simulink model "Model_V5"  (R2024b)
settings: Solver=VariableStepAuto  StartTime=0.0  StopTime=3600*12  RelTol=1e-3
undefined symbols (not defined in the file): PropsSI
libraries: fl_lib x569, SimscapeFluids_lib x61, nesl_utility x27
(part 6 of 7)

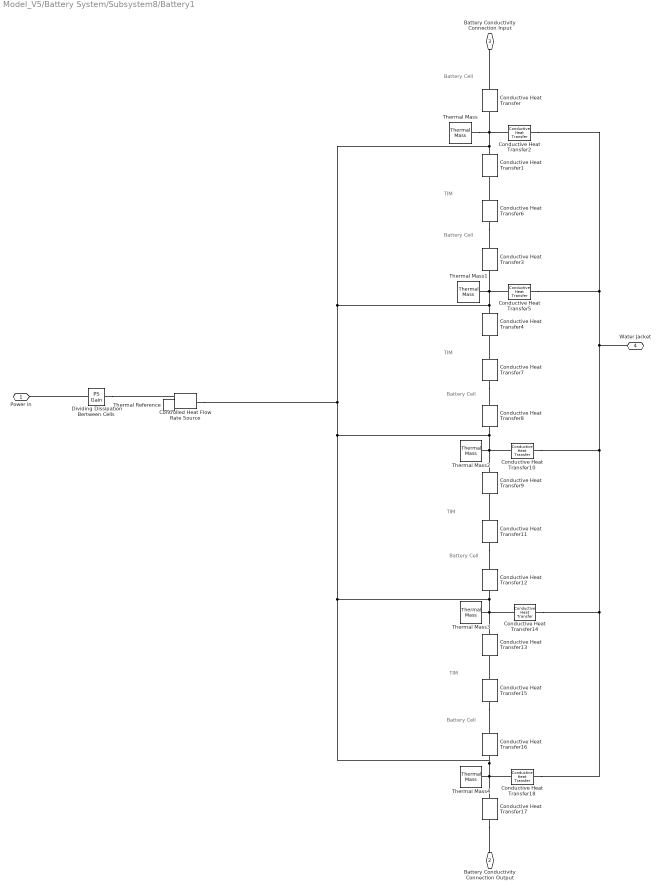
== system Model_V5/Battery System/Subsystem8/Battery1 ==
  note: TIM
  note: Battery Cell
  note: TIM
  note: Battery Cell
  note: TIM
  note: Battery Cell
  note: TIM
  note: Battery Cell
  note: Battery Cell
  Conductive Heat Transfer{,1,3..4,8..9,12..13,16..17} (10 alike) : fl_lib/Thermal/Thermal Elements/Conductive Heat Transfer  thermal_type=foundation.enum.ConstantVariableTabulated.Constant  wall_geometry=foundation.enum.ConductionWallGeometry.Planar  area=301.5*99.7 mm^2  thickness=11.6/2 mm  d_in=0.05 m  d_out=0.1 m  L=1 m  th_cond_min=10 W/(K*m)  th_cond=19 W/(K*m)  th_cond_TLU=[413, 401, 392, 383, 371, 357, 342] W/(K*m)  temp_TLU=[200, 273, 400, 600, 800, 1000, 1200] K  T_specify=off  T_priority=None  T=0 K  T_nominal_specify=off  T_nominal_value=1  T_nominal_unit=K  Q_specify=off  Q_priority=None  Q=0 W  Q_nominal_specify=off  Q_nominal_value=1  Q_nominal_unit=W
  Conductive Heat Transfer{2,5,10,14,18} (5 alike) : fl_lib/Thermal/Thermal Elements/Conductive Heat Transfer  thermal_type=foundation.enum.ConstantVariableTabulated.Constant  wall_geometry=foundation.enum.ConductionWallGeometry.Planar  area=(2*(301.1*11.6)) + (2*(99.9*11.7)) mm^2  thickness=0.003 in  d_in=0.05 m  d_out=0.1 m  L=1 m  th_cond_min=10 W/(K*m)  th_cond=1.38 W/(K*m)  th_cond_TLU=[413, 401, 392, 383, 371, 357, 342] W/(K*m)  temp_TLU=[200, 273, 400, 600, 800, 1000, 1200] K  T_specify=off  T_priority=None  T=0 K  T_nominal_specify=off  T_nominal_value=1  T_nominal_unit=K  Q_specify=off  Q_priority=None  Q=0 W  Q_nominal_specify=off  Q_nominal_value=1  Q_nominal_unit=W
  Conductive Heat Transfer{6..7,11,15} (4 alike) : fl_lib/Thermal/Thermal Elements/Conductive Heat Transfer  thermal_type=foundation.enum.ConstantVariableTabulated.Constant  wall_geometry=foundation.enum.ConductionWallGeometry.Planar  area=301.5*99.7 mm^2  thickness=0.003 in  d_in=0.05 m  d_out=0.1 m  L=1 m  th_cond_min=10 W/(K*m)  th_cond=8.89 W/(K*m)  th_cond_TLU=[413, 401, 392, 383, 371, 357, 342] W/(K*m)  temp_TLU=[200, 273, 400, 600, 800, 1000, 1200] K  T_specify=off  T_priority=None  T=0 K  T_nominal_specify=off  T_nominal_value=1  T_nominal_unit=K  Q_specify=off  Q_priority=None  Q=0 W  Q_nominal_specify=off  Q_nominal_value=1  Q_nominal_unit=W
  Controlled Heat Flow Rate Source : fl_lib/Thermal/Thermal Sources/Controlled Heat Flow Rate Source
  Dividing Dissipation Bertween Cells : fl_lib/Physical Signals/Functions/PS Gain  gain=1/5
  Thermal Mass{,1..4} (5 alike) : fl_lib/Thermal/Thermal Elements/Thermal Mass  mass_type=foundation.enum.constant_variable.constant  mass=740 g  sp_heat=1040 J/(K*kg)  mass_min=1e-6 kg  num_ports=foundation.enum.numPorts2.one  m_specify=off  m_priority=High  m=1 kg  m_nominal_specify=off  m_nominal_value=1  m_nominal_unit=kg  T_specify=on  T_priority=Low  T=292 K  T_nominal_specify=off  T_nominal_value=1  T_nominal_unit=K  Q_specify=off  Q_priority=None  Q=0 W  Q_nominal_specify=off  Q_nominal_value=1  Q_nominal_unit=W
  Thermal Reference : fl_lib/Thermal/Thermal Elements/Thermal Reference
  Power in : PMIOPort  Side=Left
  Battery Conductivity Connection Output : PMIOPort  Port=2  Side=Left
  Battery Conductivity Connection Input : PMIOPort  Port=3  Side=Right
  Water Jacket : PMIOPort  Port=4  Side=Right
  connections:
  Conductive Heat Transfer7/RConn1 -- Conductive Heat Transfer8/LConn1
  Conductive Heat Transfer17/RConn1 -- Battery Conductivity Connection Output/RConn1
  Conductive Heat Transfer6/RConn1 -- Conductive Heat Transfer3/LConn1
  Conductive Heat Transfer18/RConn1 -- Conductive Heat Transfer14/RConn1 -- Conductive Heat Transfer10/RConn1 -- Conductive Heat Transfer2/RConn1 -- Conductive Heat Transfer5/RConn1 -- Water Jacket/RConn1
  Conductive Heat Transfer8/RConn1 -- Conductive Heat Transfer10/LConn1 -- Thermal Mass2/LConn1 -- Conductive Heat Transfer9/LConn1 -- Conductive Heat Transfer12/RConn1 -- Thermal Mass3/LConn1 -- Conductive Heat Transfer14/LConn1 -- Conductive Heat Transfer13/LConn1 -- Conductive Heat Transfer18/LConn1 -- Thermal Mass4/LConn1 -- Conductive Heat Transfer17/LConn1 -- Conductive Heat Transfer16/RConn1 -- Conductive Heat Transfer2/LConn1 -- Thermal Mass/LConn1 -- Conductive Heat Transfer/RConn1 -- Conductive Heat Transfer1/LConn1 -- Conductive Heat Transfer5/LConn1 -- Thermal Mass1/LConn1 -- Conductive Heat Transfer3/RConn1 -- Conductive Heat Transfer4/LConn1 -- Controlled Heat Flow Rate Source/LConn1
  Conductive Heat Transfer15/LConn1 -- Conductive Heat Transfer13/RConn1
  Conductive Heat Transfer11/LConn1 -- Conductive Heat Transfer9/RConn1
  Conductive Heat Transfer7/LConn1 -- Conductive Heat Transfer4/RConn1
  Conductive Heat Transfer11/RConn1 -- Conductive Heat Transfer12/LConn1
  Conductive Heat Transfer6/LConn1 -- Conductive Heat Transfer1/RConn1
  Conductive Heat Transfer15/RConn1 -- Conductive Heat Transfer16/LConn1
  Conductive Heat Transfer/LConn1 -- Battery Conductivity Connection Input/RConn1
  Thermal Reference/LConn1 -- Controlled Heat Flow Rate Source/RConn2
  Dividing Dissipation Bertween Cells/LConn1 -- Power in/RConn1
  Dividing Dissipation Bertween Cells/RConn1 -- Controlled Heat Flow Rate Source/RConn1

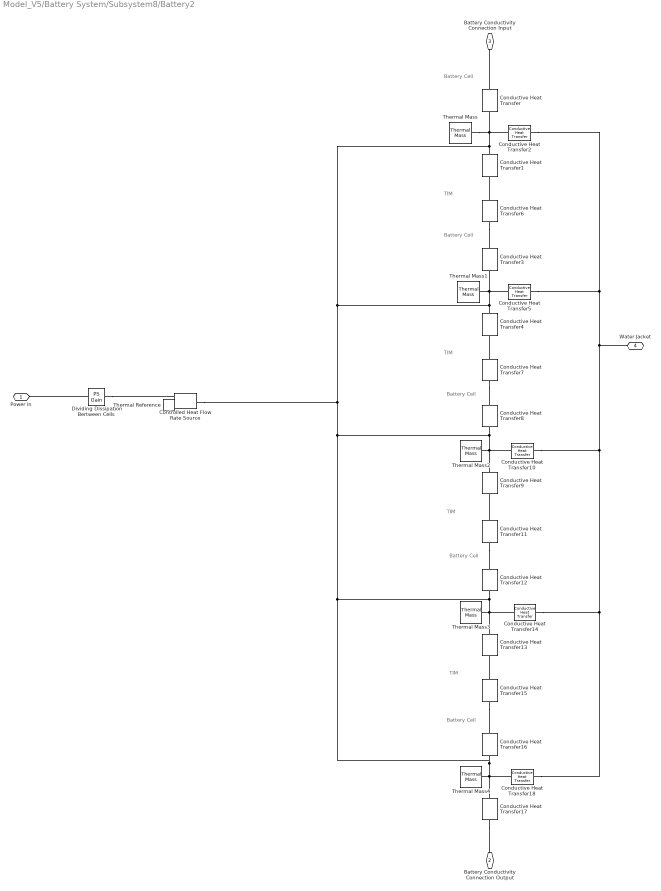
== system Model_V5/Battery System/Subsystem8/Battery2 ==
  note: TIM
  note: Battery Cell
  note: TIM
  note: Battery Cell
  note: TIM
  note: Battery Cell
  note: TIM
  note: Battery Cell
  note: Battery Cell
  Conductive Heat Transfer{,1,3..4,8..9,12..13,16..17} (10 alike) : fl_lib/Thermal/Thermal Elements/Conductive Heat Transfer  thermal_type=foundation.enum.ConstantVariableTabulated.Constant  wall_geometry=foundation.enum.ConductionWallGeometry.Planar  area=301.5*99.7 mm^2  thickness=11.6/2 mm  d_in=0.05 m  d_out=0.1 m  L=1 m  th_cond_min=10 W/(K*m)  th_cond=19 W/(K*m)  th_cond_TLU=[413, 401, 392, 383, 371, 357, 342] W/(K*m)  temp_TLU=[200, 273, 400, 600, 800, 1000, 1200] K  T_specify=off  T_priority=None  T=0 K  T_nominal_specify=off  T_nominal_value=1  T_nominal_unit=K  Q_specify=off  Q_priority=None  Q=0 W  Q_nominal_specify=off  Q_nominal_value=1  Q_nominal_unit=W
  Conductive Heat Transfer{2,5,10,14,18} (5 alike) : fl_lib/Thermal/Thermal Elements/Conductive Heat Transfer  thermal_type=foundation.enum.ConstantVariableTabulated.Constant  wall_geometry=foundation.enum.ConductionWallGeometry.Planar  area=(2*(301.1*11.6)) + (2*(99.9*11.7)) mm^2  thickness=0.003 in  d_in=0.05 m  d_out=0.1 m  L=1 m  th_cond_min=10 W/(K*m)  th_cond=1.38 W/(K*m)  th_cond_TLU=[413, 401, 392, 383, 371, 357, 342] W/(K*m)  temp_TLU=[200, 273, 400, 600, 800, 1000, 1200] K  T_specify=off  T_priority=None  T=0 K  T_nominal_specify=off  T_nominal_value=1  T_nominal_unit=K  Q_specify=off  Q_priority=None  Q=0 W  Q_nominal_specify=off  Q_nominal_value=1  Q_nominal_unit=W
  Conductive Heat Transfer{6..7,11,15} (4 alike) : fl_lib/Thermal/Thermal Elements/Conductive Heat Transfer  thermal_type=foundation.enum.ConstantVariableTabulated.Constant  wall_geometry=foundation.enum.ConductionWallGeometry.Planar  area=301.5*99.7 mm^2  thickness=0.003 in  d_in=0.05 m  d_out=0.1 m  L=1 m  th_cond_min=10 W/(K*m)  th_cond=8.89 W/(K*m)  th_cond_TLU=[413, 401, 392, 383, 371, 357, 342] W/(K*m)  temp_TLU=[200, 273, 400, 600, 800, 1000, 1200] K  T_specify=off  T_priority=None  T=0 K  T_nominal_specify=off  T_nominal_value=1  T_nominal_unit=K  Q_specify=off  Q_priority=None  Q=0 W  Q_nominal_specify=off  Q_nominal_value=1  Q_nominal_unit=W
  Controlled Heat Flow Rate Source : fl_lib/Thermal/Thermal Sources/Controlled Heat Flow Rate Source
  Dividing Dissipation Bertween Cells : fl_lib/Physical Signals/Functions/PS Gain  gain=1/5
  Thermal Mass{,1..4} (5 alike) : fl_lib/Thermal/Thermal Elements/Thermal Mass  mass_type=foundation.enum.constant_variable.constant  mass=740 g  sp_heat=1040 J/(K*kg)  mass_min=1e-6 kg  num_ports=foundation.enum.numPorts2.one  m_specify=off  m_priority=High  m=1 kg  m_nominal_specify=off  m_nominal_value=1  m_nominal_unit=kg  T_specify=on  T_priority=Low  T=292 K  T_nominal_specify=off  T_nominal_value=1  T_nominal_unit=K  Q_specify=off  Q_priority=None  Q=0 W  Q_nominal_specify=off  Q_nominal_value=1  Q_nominal_unit=W
  Thermal Reference : fl_lib/Thermal/Thermal Elements/Thermal Reference
  Power in : PMIOPort  Side=Left
  Battery Conductivity Connection Output : PMIOPort  Port=2  Side=Left
  Battery Conductivity Connection Input : PMIOPort  Port=3  Side=Right
  Water Jacket : PMIOPort  Port=4  Side=Right
  connections:
  Conductive Heat Transfer7/RConn1 -- Conductive Heat Transfer8/LConn1
  Conductive Heat Transfer17/RConn1 -- Battery Conductivity Connection Output/RConn1
  Conductive Heat Transfer6/RConn1 -- Conductive Heat Transfer3/LConn1
  Conductive Heat Transfer18/RConn1 -- Conductive Heat Transfer14/RConn1 -- Conductive Heat Transfer10/RConn1 -- Conductive Heat Transfer2/RConn1 -- Conductive Heat Transfer5/RConn1 -- Water Jacket/RConn1
  Conductive Heat Transfer8/RConn1 -- Conductive Heat Transfer10/LConn1 -- Thermal Mass2/LConn1 -- Conductive Heat Transfer9/LConn1 -- Conductive Heat Transfer12/RConn1 -- Thermal Mass3/LConn1 -- Conductive Heat Transfer14/LConn1 -- Conductive Heat Transfer13/LConn1 -- Conductive Heat Transfer18/LConn1 -- Thermal Mass4/LConn1 -- Conductive Heat Transfer17/LConn1 -- Conductive Heat Transfer16/RConn1 -- Conductive Heat Transfer2/LConn1 -- Thermal Mass/LConn1 -- Conductive Heat Transfer/RConn1 -- Conductive Heat Transfer1/LConn1 -- Conductive Heat Transfer5/LConn1 -- Thermal Mass1/LConn1 -- Conductive Heat Transfer3/RConn1 -- Conductive Heat Transfer4/LConn1 -- Controlled Heat Flow Rate Source/LConn1
  Conductive Heat Transfer15/LConn1 -- Conductive Heat Transfer13/RConn1
  Conductive Heat Transfer11/LConn1 -- Conductive Heat Transfer9/RConn1
  Conductive Heat Transfer7/LConn1 -- Conductive Heat Transfer4/RConn1
  Conductive Heat Transfer11/RConn1 -- Conductive Heat Transfer12/LConn1
  Conductive Heat Transfer6/LConn1 -- Conductive Heat Transfer1/RConn1
  Conductive Heat Transfer15/RConn1 -- Conductive Heat Transfer16/LConn1
  Conductive Heat Transfer/LConn1 -- Battery Conductivity Connection Input/RConn1
  Thermal Reference/LConn1 -- Controlled Heat Flow Rate Source/RConn2
  Dividing Dissipation Bertween Cells/LConn1 -- Power in/RConn1
  Dividing Dissipation Bertween Cells/RConn1 -- Controlled Heat Flow Rate Source/RConn1

== system Model_V5/Battery System/Subsystem8/Battery3 ==
  note: TIM
  note: Battery Cell
  note: TIM
  note: Battery Cell
  note: TIM
  note: Battery Cell
  note: TIM
  note: Battery Cell
  note: Battery Cell
  Conductive Heat Transfer{,1,3..4,8..9,12..13,16} (9 alike) : fl_lib/Thermal/Thermal Elements/Conductive Heat Transfer  thermal_type=foundation.enum.ConstantVariableTabulated.Constant  wall_geometry=foundation.enum.ConductionWallGeometry.Planar  area=301.5*99.7 mm^2  thickness=11.6/2 mm  d_in=0.05 m  d_out=0.1 m  L=1 m  th_cond_min=10 W/(K*m)  th_cond=19 W/(K*m)  th_cond_TLU=[413, 401, 392, 383, 371, 357, 342] W/(K*m)  temp_TLU=[200, 273, 400, 600, 800, 1000, 1200] K  T_specify=off  T_priority=None  T=0 K  T_nominal_specify=off  T_nominal_value=1  T_nominal_unit=K  Q_specify=off  Q_priority=None  Q=0 W  Q_nominal_specify=off  Q_nominal_value=1  Q_nominal_unit=W
  Conductive Heat Transfer{2,5,10,14,18} (5 alike) : fl_lib/Thermal/Thermal Elements/Conductive Heat Transfer  thermal_type=foundation.enum.ConstantVariableTabulated.Constant  wall_geometry=foundation.enum.ConductionWallGeometry.Planar  area=(2*(301.1*11.6)) + (2*(99.9*11.7)) mm^2  thickness=0.003 in  d_in=0.05 m  d_out=0.1 m  L=1 m  th_cond_min=10 W/(K*m)  th_cond=1.38 W/(K*m)  th_cond_TLU=[413, 401, 392, 383, 371, 357, 342] W/(K*m)  temp_TLU=[200, 273, 400, 600, 800, 1000, 1200] K  T_specify=off  T_priority=None  T=0 K  T_nominal_specify=off  T_nominal_value=1  T_nominal_unit=K  Q_specify=off  Q_priority=None  Q=0 W  Q_nominal_specify=off  Q_nominal_value=1  Q_nominal_unit=W
  Conductive Heat Transfer{6..7,11,15} (4 alike) : fl_lib/Thermal/Thermal Elements/Conductive Heat Transfer  thermal_type=foundation.enum.ConstantVariableTabulated.Constant  wall_geometry=foundation.enum.ConductionWallGeometry.Planar  area=301.5*99.7 mm^2  thickness=0.003 in  d_in=0.05 m  d_out=0.1 m  L=1 m  th_cond_min=10 W/(K*m)  th_cond=8.89 W/(K*m)  th_cond_TLU=[413, 401, 392, 383, 371, 357, 342] W/(K*m)  temp_TLU=[200, 273, 400, 600, 800, 1000, 1200] K  T_specify=off  T_priority=None  T=0 K  T_nominal_specify=off  T_nominal_value=1  T_nominal_unit=K  Q_specify=off  Q_priority=None  Q=0 W  Q_nominal_specify=off  Q_nominal_value=1  Q_nominal_unit=W
  Controlled Heat Flow Rate Source : fl_lib/Thermal/Thermal Sources/Controlled Heat Flow Rate Source
  Dividing Dissipation Bertween Cells : fl_lib/Physical Signals/Functions/PS Gain  gain=1/5
  Thermal Mass{,1..4} (5 alike) : fl_lib/Thermal/Thermal Elements/Thermal Mass  mass_type=foundation.enum.constant_variable.constant  mass=740 g  sp_heat=1040 J/(K*kg)  mass_min=1e-6 kg  num_ports=foundation.enum.numPorts2.one  m_specify=off  m_priority=High  m=1 kg  m_nominal_specify=off  m_nominal_value=1  m_nominal_unit=kg  T_specify=on  T_priority=Low  T=292 K  T_nominal_specify=off  T_nominal_value=1  T_nominal_unit=K  Q_specify=off  Q_priority=None  Q=0 W  Q_nominal_specify=off  Q_nominal_value=1  Q_nominal_unit=W
  Thermal Reference : fl_lib/Thermal/Thermal Elements/Thermal Reference
  Power in : PMIOPort  Side=Left
  Battery Conductivity Connection Input : PMIOPort  Port=2  Side=Right
  Water Jacket : PMIOPort  Port=3  Side=Right
  connections:
  Conductive Heat Transfer7/RConn1 -- Conductive Heat Transfer8/LConn1
  Conductive Heat Transfer6/RConn1 -- Conductive Heat Transfer3/LConn1
  Conductive Heat Transfer18/RConn1 -- Conductive Heat Transfer14/RConn1 -- Conductive Heat Transfer10/RConn1 -- Conductive Heat Transfer2/RConn1 -- Conductive Heat Transfer5/RConn1 -- Water Jacket/RConn1
  Conductive Heat Transfer8/RConn1 -- Conductive Heat Transfer10/LConn1 -- Thermal Mass2/LConn1 -- Conductive Heat Transfer9/LConn1 -- Conductive Heat Transfer12/RConn1 -- Thermal Mass3/LConn1 -- Conductive Heat Transfer14/LConn1 -- Conductive Heat Transfer13/LConn1 -- Conductive Heat Transfer18/LConn1 -- Thermal Mass4/LConn1 -- Conductive Heat Transfer16/RConn1 -- Conductive Heat Transfer2/LConn1 -- Thermal Mass/LConn1 -- Conductive Heat Transfer/RConn1 -- Conductive Heat Transfer1/LConn1 -- Conductive Heat Transfer5/LConn1 -- Thermal Mass1/LConn1 -- Conductive Heat Transfer3/RConn1 -- Conductive Heat Transfer4/LConn1 -- Controlled Heat Flow Rate Source/LConn1
  Conductive Heat Transfer15/LConn1 -- Conductive Heat Transfer13/RConn1
  Conductive Heat Transfer11/LConn1 -- Conductive Heat Transfer9/RConn1
  Conductive Heat Transfer7/LConn1 -- Conductive Heat Transfer4/RConn1
  Conductive Heat Transfer11/RConn1 -- Conductive Heat Transfer12/LConn1
  Conductive Heat Transfer6/LConn1 -- Conductive Heat Transfer1/RConn1
  Conductive Heat Transfer15/RConn1 -- Conductive Heat Transfer16/LConn1
  Conductive Heat Transfer/LConn1 -- Battery Conductivity Connection Input/RConn1
  Thermal Reference/LConn1 -- Controlled Heat Flow Rate Source/RConn2
  Dividing Dissipation Bertween Cells/LConn1 -- Power in/RConn1
  Dividing Dissipation Bertween Cells/RConn1 -- Controlled Heat Flow Rate Source/RConn1

== system Model_V5/Battery System/Subsystem8/Battery4 ==
  note: TIM
  note: Battery Cell
  note: TIM
  note: Battery Cell
  note: TIM
  note: Battery Cell
  note: TIM
  note: Battery Cell
  note: Battery Cell
  Conductive Heat Transfer{1,3..4,8..9,12..13,16..17} (9 alike) : fl_lib/Thermal/Thermal Elements/Conductive Heat Transfer  thermal_type=foundation.enum.ConstantVariableTabulated.Constant  wall_geometry=foundation.enum.ConductionWallGeometry.Planar  area=301.5*99.7 mm^2  thickness=11.6/2 mm  d_in=0.05 m  d_out=0.1 m  L=1 m  th_cond_min=10 W/(K*m)  th_cond=19 W/(K*m)  th_cond_TLU=[413, 401, 392, 383, 371, 357, 342] W/(K*m)  temp_TLU=[200, 273, 400, 600, 800, 1000, 1200] K  T_specify=off  T_priority=None  T=0 K  T_nominal_specify=off  T_nominal_value=1  T_nominal_unit=K  Q_specify=off  Q_priority=None  Q=0 W  Q_nominal_specify=off  Q_nominal_value=1  Q_nominal_unit=W
  Conductive Heat Transfer{2,5,10,14,18} (5 alike) : fl_lib/Thermal/Thermal Elements/Conductive Heat Transfer  thermal_type=foundation.enum.ConstantVariableTabulated.Constant  wall_geometry=foundation.enum.ConductionWallGeometry.Planar  area=(2*(301.1*11.6)) + (2*(99.9*11.7)) mm^2  thickness=0.003 in  d_in=0.05 m  d_out=0.1 m  L=1 m  th_cond_min=10 W/(K*m)  th_cond=1.38 W/(K*m)  th_cond_TLU=[413, 401, 392, 383, 371, 357, 342] W/(K*m)  temp_TLU=[200, 273, 400, 600, 800, 1000, 1200] K  T_specify=off  T_priority=None  T=0 K  T_nominal_specify=off  T_nominal_value=1  T_nominal_unit=K  Q_specify=off  Q_priority=None  Q=0 W  Q_nominal_specify=off  Q_nominal_value=1  Q_nominal_unit=W
  Conductive Heat Transfer{6..7,11,15} (4 alike) : fl_lib/Thermal/Thermal Elements/Conductive Heat Transfer  thermal_type=foundation.enum.ConstantVariableTabulated.Constant  wall_geometry=foundation.enum.ConductionWallGeometry.Planar  area=301.5*99.7 mm^2  thickness=0.003 in  d_in=0.05 m  d_out=0.1 m  L=1 m  th_cond_min=10 W/(K*m)  th_cond=8.89 W/(K*m)  th_cond_TLU=[413, 401, 392, 383, 371, 357, 342] W/(K*m)  temp_TLU=[200, 273, 400, 600, 800, 1000, 1200] K  T_specify=off  T_priority=None  T=0 K  T_nominal_specify=off  T_nominal_value=1  T_nominal_unit=K  Q_specify=off  Q_priority=None  Q=0 W  Q_nominal_specify=off  Q_nominal_value=1  Q_nominal_unit=W
  Controlled Heat Flow Rate Source : fl_lib/Thermal/Thermal Sources/Controlled Heat Flow Rate Source
  Dividing Dissipation Bertween Cells : fl_lib/Physical Signals/Functions/PS Gain  gain=1/5
  Thermal Mass{,1..4} (5 alike) : fl_lib/Thermal/Thermal Elements/Thermal Mass  mass_type=foundation.enum.constant_variable.constant  mass=740 g  sp_heat=1040 J/(K*kg)  mass_min=1e-6 kg  num_ports=foundation.enum.numPorts2.one  m_specify=off  m_priority=High  m=1 kg  m_nominal_specify=off  m_nominal_value=1  m_nominal_unit=kg  T_specify=on  T_priority=Low  T=292 K  T_nominal_specify=off  T_nominal_value=1  T_nominal_unit=K  Q_specify=off  Q_priority=None  Q=0 W  Q_nominal_specify=off  Q_nominal_value=1  Q_nominal_unit=W
  Thermal Reference : fl_lib/Thermal/Thermal Elements/Thermal Reference
  Power in : PMIOPort  Side=Left
  Water Jacket : PMIOPort  Port=2  Side=Right
  Battery Conductivity Connection Output : PMIOPort  Port=3  Side=Right
  connections:
  Conductive Heat Transfer7/RConn1 -- Conductive Heat Transfer8/LConn1
  Conductive Heat Transfer17/RConn1 -- Battery Conductivity Connection Output/RConn1
  Conductive Heat Transfer6/RConn1 -- Conductive Heat Transfer3/LConn1
  Conductive Heat Transfer18/RConn1 -- Conductive Heat Transfer14/RConn1 -- Conductive Heat Transfer10/RConn1 -- Conductive Heat Transfer2/RConn1 -- Conductive Heat Transfer5/RConn1 -- Water Jacket/RConn1
  Conductive Heat Transfer8/RConn1 -- Conductive Heat Transfer10/LConn1 -- Thermal Mass2/LConn1 -- Conductive Heat Transfer9/LConn1 -- Conductive Heat Transfer12/RConn1 -- Thermal Mass3/LConn1 -- Conductive Heat Transfer14/LConn1 -- Conductive Heat Transfer13/LConn1 -- Conductive Heat Transfer18/LConn1 -- Thermal Mass4/LConn1 -- Conductive Heat Transfer17/LConn1 -- Conductive Heat Transfer16/RConn1 -- Conductive Heat Transfer2/LConn1 -- Thermal Mass/LConn1 -- Conductive Heat Transfer1/LConn1 -- Conductive Heat Transfer5/LConn1 -- Thermal Mass1/LConn1 -- Conductive Heat Transfer3/RConn1 -- Conductive Heat Transfer4/LConn1 -- Controlled Heat Flow Rate Source/LConn1
  Conductive Heat Transfer15/LConn1 -- Conductive Heat Transfer13/RConn1
  Conductive Heat Transfer11/LConn1 -- Conductive Heat Transfer9/RConn1
  Conductive Heat Transfer7/LConn1 -- Conductive Heat Transfer4/RConn1
  Conductive Heat Transfer11/RConn1 -- Conductive Heat Transfer12/LConn1
  Conductive Heat Transfer6/LConn1 -- Conductive Heat Transfer1/RConn1
  Conductive Heat Transfer15/RConn1 -- Conductive Heat Transfer16/LConn1
  Thermal Reference/LConn1 -- Controlled Heat Flow Rate Source/RConn2
  Dividing Dissipation Bertween Cells/LConn1 -- Power in/RConn1
  Dividing Dissipation Bertween Cells/RConn1 -- Controlled Heat Flow Rate Source/RConn1

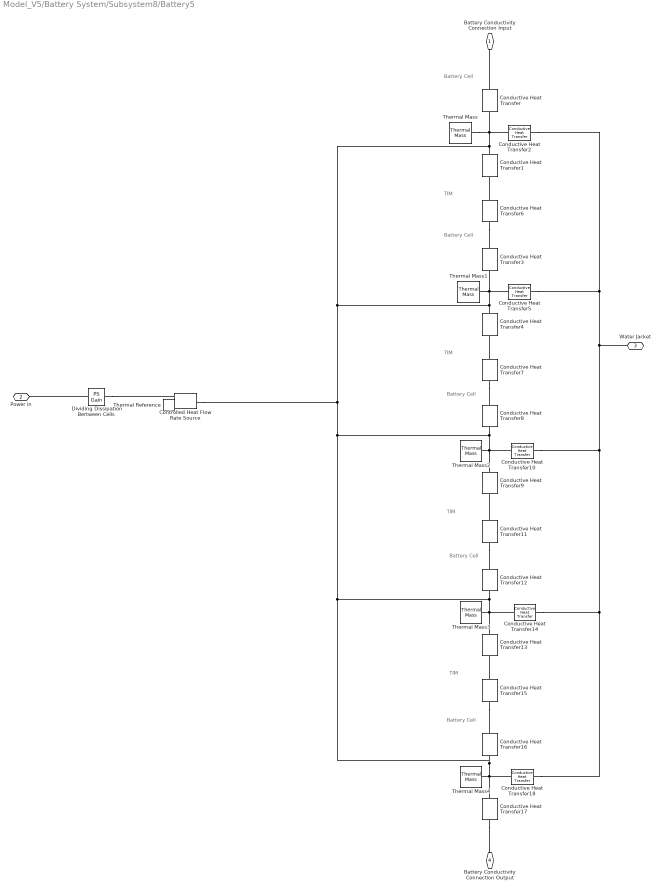
== system Model_V5/Battery System/Subsystem8/Battery5 ==
  note: TIM
  note: Battery Cell
  note: TIM
  note: Battery Cell
  note: TIM
  note: Battery Cell
  note: TIM
  note: Battery Cell
  note: Battery Cell
  Conductive Heat Transfer{,1,3..4,8..9,12..13,16..17} (10 alike) : fl_lib/Thermal/Thermal Elements/Conductive Heat Transfer  thermal_type=foundation.enum.ConstantVariableTabulated.Constant  wall_geometry=foundation.enum.ConductionWallGeometry.Planar  area=301.5*99.7 mm^2  thickness=11.6/2 mm  d_in=0.05 m  d_out=0.1 m  L=1 m  th_cond_min=10 W/(K*m)  th_cond=19 W/(K*m)  th_cond_TLU=[413, 401, 392, 383, 371, 357, 342] W/(K*m)  temp_TLU=[200, 273, 400, 600, 800, 1000, 1200] K  T_specify=off  T_priority=None  T=0 K  T_nominal_specify=off  T_nominal_value=1  T_nominal_unit=K  Q_specify=off  Q_priority=None  Q=0 W  Q_nominal_specify=off  Q_nominal_value=1  Q_nominal_unit=W
  Conductive Heat Transfer{2,5,10,14,18} (5 alike) : fl_lib/Thermal/Thermal Elements/Conductive Heat Transfer  thermal_type=foundation.enum.ConstantVariableTabulated.Constant  wall_geometry=foundation.enum.ConductionWallGeometry.Planar  area=(2*(301.1*11.6)) + (2*(99.9*11.7)) mm^2  thickness=0.003 in  d_in=0.05 m  d_out=0.1 m  L=1 m  th_cond_min=10 W/(K*m)  th_cond=1.38 W/(K*m)  th_cond_TLU=[413, 401, 392, 383, 371, 357, 342] W/(K*m)  temp_TLU=[200, 273, 400, 600, 800, 1000, 1200] K  T_specify=off  T_priority=None  T=0 K  T_nominal_specify=off  T_nominal_value=1  T_nominal_unit=K  Q_specify=off  Q_priority=None  Q=0 W  Q_nominal_specify=off  Q_nominal_value=1  Q_nominal_unit=W
  Conductive Heat Transfer{6..7,11,15} (4 alike) : fl_lib/Thermal/Thermal Elements/Conductive Heat Transfer  thermal_type=foundation.enum.ConstantVariableTabulated.Constant  wall_geometry=foundation.enum.ConductionWallGeometry.Planar  area=301.5*99.7 mm^2  thickness=0.003 in  d_in=0.05 m  d_out=0.1 m  L=1 m  th_cond_min=10 W/(K*m)  th_cond=8.89 W/(K*m)  th_cond_TLU=[413, 401, 392, 383, 371, 357, 342] W/(K*m)  temp_TLU=[200, 273, 400, 600, 800, 1000, 1200] K  T_specify=off  T_priority=None  T=0 K  T_nominal_specify=off  T_nominal_value=1  T_nominal_unit=K  Q_specify=off  Q_priority=None  Q=0 W  Q_nominal_specify=off  Q_nominal_value=1  Q_nominal_unit=W
  Controlled Heat Flow Rate Source : fl_lib/Thermal/Thermal Sources/Controlled Heat Flow Rate Source
  Dividing Dissipation Bertween Cells : fl_lib/Physical Signals/Functions/PS Gain  gain=1/5
  Thermal Mass{,1..4} (5 alike) : fl_lib/Thermal/Thermal Elements/Thermal Mass  mass_type=foundation.enum.constant_variable.constant  mass=740 g  sp_heat=1040 J/(K*kg)  mass_min=1e-6 kg  num_ports=foundation.enum.numPorts2.one  m_specify=off  m_priority=High  m=1 kg  m_nominal_specify=off  m_nominal_value=1  m_nominal_unit=kg  T_specify=on  T_priority=Low  T=292 K  T_nominal_specify=off  T_nominal_value=1  T_nominal_unit=K  Q_specify=off  Q_priority=None  Q=0 W  Q_nominal_specify=off  Q_nominal_value=1  Q_nominal_unit=W
  Thermal Reference : fl_lib/Thermal/Thermal Elements/Thermal Reference
  Battery Conductivity Connection Input : PMIOPort  Side=Left
  Power in : PMIOPort  Port=2  Side=Left
  Water Jacket : PMIOPort  Port=3  Side=Right
  Battery Conductivity Connection Output : PMIOPort  Port=4  Side=Right
  connections:
  Conductive Heat Transfer7/RConn1 -- Conductive Heat Transfer8/LConn1
  Conductive Heat Transfer17/RConn1 -- Battery Conductivity Connection Output/RConn1
  Conductive Heat Transfer6/RConn1 -- Conductive Heat Transfer3/LConn1
  Conductive Heat Transfer18/RConn1 -- Conductive Heat Transfer14/RConn1 -- Conductive Heat Transfer10/RConn1 -- Conductive Heat Transfer2/RConn1 -- Conductive Heat Transfer5/RConn1 -- Water Jacket/RConn1
  Conductive Heat Transfer8/RConn1 -- Conductive Heat Transfer10/LConn1 -- Thermal Mass2/LConn1 -- Conductive Heat Transfer9/LConn1 -- Conductive Heat Transfer12/RConn1 -- Thermal Mass3/LConn1 -- Conductive Heat Transfer14/LConn1 -- Conductive Heat Transfer13/LConn1 -- Conductive Heat Transfer18/LConn1 -- Thermal Mass4/LConn1 -- Conductive Heat Transfer17/LConn1 -- Conductive Heat Transfer16/RConn1 -- Conductive Heat Transfer2/LConn1 -- Thermal Mass/LConn1 -- Conductive Heat Transfer/RConn1 -- Conductive Heat Transfer1/LConn1 -- Conductive Heat Transfer5/LConn1 -- Thermal Mass1/LConn1 -- Conductive Heat Transfer3/RConn1 -- Conductive Heat Transfer4/LConn1 -- Controlled Heat Flow Rate Source/LConn1
  Conductive Heat Transfer15/LConn1 -- Conductive Heat Transfer13/RConn1
  Conductive Heat Transfer11/LConn1 -- Conductive Heat Transfer9/RConn1
  Conductive Heat Transfer7/LConn1 -- Conductive Heat Transfer4/RConn1
  Conductive Heat Transfer11/RConn1 -- Conductive Heat Transfer12/LConn1
  Conductive Heat Transfer6/LConn1 -- Conductive Heat Transfer1/RConn1
  Conductive Heat Transfer15/RConn1 -- Conductive Heat Transfer16/LConn1
  Conductive Heat Transfer/LConn1 -- Battery Conductivity Connection Input/RConn1
  Thermal Reference/LConn1 -- Controlled Heat Flow Rate Source/RConn2
  Dividing Dissipation Bertween Cells/LConn1 -- Power in/RConn1
  Dividing Dissipation Bertween Cells/RConn1 -- Controlled Heat Flow Rate Source/RConn1

== system Model_V5/Battery System/Subsystem8/Battery6 ==
  note: TIM
  note: Battery Cell
  note: TIM
  note: Battery Cell
  note: TIM
  note: Battery Cell
  note: TIM
  note: Battery Cell
  note: Battery Cell
  Conductive Heat Transfer{,1,3..4,8..9,12..13,16..17} (10 alike) : fl_lib/Thermal/Thermal Elements/Conductive Heat Transfer  thermal_type=foundation.enum.ConstantVariableTabulated.Constant  wall_geometry=foundation.enum.ConductionWallGeometry.Planar  area=301.5*99.7 mm^2  thickness=11.6/2 mm  d_in=0.05 m  d_out=0.1 m  L=1 m  th_cond_min=10 W/(K*m)  th_cond=19 W/(K*m)  th_cond_TLU=[413, 401, 392, 383, 371, 357, 342] W/(K*m)  temp_TLU=[200, 273, 400, 600, 800, 1000, 1200] K  T_specify=off  T_priority=None  T=0 K  T_nominal_specify=off  T_nominal_value=1  T_nominal_unit=K  Q_specify=off  Q_priority=None  Q=0 W  Q_nominal_specify=off  Q_nominal_value=1  Q_nominal_unit=W
  Conductive Heat Transfer{2,5,10,14,18} (5 alike) : fl_lib/Thermal/Thermal Elements/Conductive Heat Transfer  thermal_type=foundation.enum.ConstantVariableTabulated.Constant  wall_geometry=foundation.enum.ConductionWallGeometry.Planar  area=(2*(301.1*11.6)) + (2*(99.9*11.7)) mm^2  thickness=0.003 in  d_in=0.05 m  d_out=0.1 m  L=1 m  th_cond_min=10 W/(K*m)  th_cond=1.38 W/(K*m)  th_cond_TLU=[413, 401, 392, 383, 371, 357, 342] W/(K*m)  temp_TLU=[200, 273, 400, 600, 800, 1000, 1200] K  T_specify=off  T_priority=None  T=0 K  T_nominal_specify=off  T_nominal_value=1  T_nominal_unit=K  Q_specify=off  Q_priority=None  Q=0 W  Q_nominal_specify=off  Q_nominal_value=1  Q_nominal_unit=W
  Conductive Heat Transfer{6..7,11,15} (4 alike) : fl_lib/Thermal/Thermal Elements/Conductive Heat Transfer  thermal_type=foundation.enum.ConstantVariableTabulated.Constant  wall_geometry=foundation.enum.ConductionWallGeometry.Planar  area=301.5*99.7 mm^2  thickness=0.003 in  d_in=0.05 m  d_out=0.1 m  L=1 m  th_cond_min=10 W/(K*m)  th_cond=8.89 W/(K*m)  th_cond_TLU=[413, 401, 392, 383, 371, 357, 342] W/(K*m)  temp_TLU=[200, 273, 400, 600, 800, 1000, 1200] K  T_specify=off  T_priority=None  T=0 K  T_nominal_specify=off  T_nominal_value=1  T_nominal_unit=K  Q_specify=off  Q_priority=None  Q=0 W  Q_nominal_specify=off  Q_nominal_value=1  Q_nominal_unit=W
  Controlled Heat Flow Rate Source : fl_lib/Thermal/Thermal Sources/Controlled Heat Flow Rate Source
  Dividing Dissipation Bertween Cells : fl_lib/Physical Signals/Functions/PS Gain  gain=1/5
  Thermal Mass{,1..4} (5 alike) : fl_lib/Thermal/Thermal Elements/Thermal Mass  mass_type=foundation.enum.constant_variable.constant  mass=740 g  sp_heat=1040 J/(K*kg)  mass_min=1e-6 kg  num_ports=foundation.enum.numPorts2.one  m_specify=off  m_priority=High  m=1 kg  m_nominal_specify=off  m_nominal_value=1  m_nominal_unit=kg  T_specify=on  T_priority=Low  T=292 K  T_nominal_specify=off  T_nominal_value=1  T_nominal_unit=K  Q_specify=off  Q_priority=None  Q=0 W  Q_nominal_specify=off  Q_nominal_value=1  Q_nominal_unit=W
  Thermal Reference : fl_lib/Thermal/Thermal Elements/Thermal Reference
  Battery Conductivity Connection Input : PMIOPort  Side=Left
  Power in : PMIOPort  Port=2  Side=Left
  Water Jacket : PMIOPort  Port=3  Side=Right
  Battery Conductivity Connection Output : PMIOPort  Port=4  Side=Right
  connections:
  Conductive Heat Transfer7/RConn1 -- Conductive Heat Transfer8/LConn1
  Conductive Heat Transfer17/RConn1 -- Battery Conductivity Connection Output/RConn1
  Conductive Heat Transfer6/RConn1 -- Conductive Heat Transfer3/LConn1
  Conductive Heat Transfer18/RConn1 -- Conductive Heat Transfer14/RConn1 -- Conductive Heat Transfer10/RConn1 -- Conductive Heat Transfer2/RConn1 -- Conductive Heat Transfer5/RConn1 -- Water Jacket/RConn1
  Conductive Heat Transfer8/RConn1 -- Conductive Heat Transfer10/LConn1 -- Thermal Mass2/LConn1 -- Conductive Heat Transfer9/LConn1 -- Conductive Heat Transfer12/RConn1 -- Thermal Mass3/LConn1 -- Conductive Heat Transfer14/LConn1 -- Conductive Heat Transfer13/LConn1 -- Conductive Heat Transfer18/LConn1 -- Thermal Mass4/LConn1 -- Conductive Heat Transfer17/LConn1 -- Conductive Heat Transfer16/RConn1 -- Conductive Heat Transfer2/LConn1 -- Thermal Mass/LConn1 -- Conductive Heat Transfer/RConn1 -- Conductive Heat Transfer1/LConn1 -- Conductive Heat Transfer5/LConn1 -- Thermal Mass1/LConn1 -- Conductive Heat Transfer3/RConn1 -- Conductive Heat Transfer4/LConn1 -- Controlled Heat Flow Rate Source/LConn1
  Conductive Heat Transfer15/LConn1 -- Conductive Heat Transfer13/RConn1
  Conductive Heat Transfer11/LConn1 -- Conductive Heat Transfer9/RConn1
  Conductive Heat Transfer7/LConn1 -- Conductive Heat Transfer4/RConn1
  Conductive Heat Transfer11/RConn1 -- Conductive Heat Transfer12/LConn1
  Conductive Heat Transfer6/LConn1 -- Conductive Heat Transfer1/RConn1
  Conductive Heat Transfer15/RConn1 -- Conductive Heat Transfer16/LConn1
  Conductive Heat Transfer/LConn1 -- Battery Conductivity Connection Input/RConn1
  Thermal Reference/LConn1 -- Controlled Heat Flow Rate Source/RConn2
  Dividing Dissipation Bertween Cells/LConn1 -- Power in/RConn1
  Dividing Dissipation Bertween Cells/RConn1 -- Controlled Heat Flow Rate Source/RConn1

== system Model_V5/Battery System/Subsystem8/Battery7 ==
  note: TIM
  note: Battery Cell
  note: TIM
  note: Battery Cell
  note: TIM
  note: Battery Cell
  note: TIM
  note: Battery Cell
  note: Battery Cell
  Conductive Heat Transfer{,1,3..4,8..9,12..13,16} (9 alike) : fl_lib/Thermal/Thermal Elements/Conductive Heat Transfer  thermal_type=foundation.enum.ConstantVariableTabulated.Constant  wall_geometry=foundation.enum.ConductionWallGeometry.Planar  area=301.5*99.7 mm^2  thickness=11.6/2 mm  d_in=0.05 m  d_out=0.1 m  L=1 m  th_cond_min=10 W/(K*m)  th_cond=19 W/(K*m)  th_cond_TLU=[413, 401, 392, 383, 371, 357, 342] W/(K*m)  temp_TLU=[200, 273, 400, 600, 800, 1000, 1200] K  T_specify=off  T_priority=None  T=0 K  T_nominal_specify=off  T_nominal_value=1  T_nominal_unit=K  Q_specify=off  Q_priority=None  Q=0 W  Q_nominal_specify=off  Q_nominal_value=1  Q_nominal_unit=W
  Conductive Heat Transfer{2,5,10,14,18} (5 alike) : fl_lib/Thermal/Thermal Elements/Conductive Heat Transfer  thermal_type=foundation.enum.ConstantVariableTabulated.Constant  wall_geometry=foundation.enum.ConductionWallGeometry.Planar  area=(2*(301.1*11.6)) + (2*(99.9*11.7)) mm^2  thickness=0.003 in  d_in=0.05 m  d_out=0.1 m  L=1 m  th_cond_min=10 W/(K*m)  th_cond=1.38 W/(K*m)  th_cond_TLU=[413, 401, 392, 383, 371, 357, 342] W/(K*m)  temp_TLU=[200, 273, 400, 600, 800, 1000, 1200] K  T_specify=off  T_priority=None  T=0 K  T_nominal_specify=off  T_nominal_value=1  T_nominal_unit=K  Q_specify=off  Q_priority=None  Q=0 W  Q_nominal_specify=off  Q_nominal_value=1  Q_nominal_unit=W
  Conductive Heat Transfer{6..7,11,15} (4 alike) : fl_lib/Thermal/Thermal Elements/Conductive Heat Transfer  thermal_type=foundation.enum.ConstantVariableTabulated.Constant  wall_geometry=foundation.enum.ConductionWallGeometry.Planar  area=301.5*99.7 mm^2  thickness=0.003 in  d_in=0.05 m  d_out=0.1 m  L=1 m  th_cond_min=10 W/(K*m)  th_cond=8.89 W/(K*m)  th_cond_TLU=[413, 401, 392, 383, 371, 357, 342] W/(K*m)  temp_TLU=[200, 273, 400, 600, 800, 1000, 1200] K  T_specify=off  T_priority=None  T=0 K  T_nominal_specify=off  T_nominal_value=1  T_nominal_unit=K  Q_specify=off  Q_priority=None  Q=0 W  Q_nominal_specify=off  Q_nominal_value=1  Q_nominal_unit=W
  Controlled Heat Flow Rate Source : fl_lib/Thermal/Thermal Sources/Controlled Heat Flow Rate Source
  Dividing Dissipation Bertween Cells : fl_lib/Physical Signals/Functions/PS Gain  gain=1/5
  Thermal Mass{,1..4} (5 alike) : fl_lib/Thermal/Thermal Elements/Thermal Mass  mass_type=foundation.enum.constant_variable.constant  mass=740 g  sp_heat=1040 J/(K*kg)  mass_min=1e-6 kg  num_ports=foundation.enum.numPorts2.one  m_specify=off  m_priority=High  m=1 kg  m_nominal_specify=off  m_nominal_value=1  m_nominal_unit=kg  T_specify=on  T_priority=Low  T=292 K  T_nominal_specify=off  T_nominal_value=1  T_nominal_unit=K  Q_specify=off  Q_priority=None  Q=0 W  Q_nominal_specify=off  Q_nominal_value=1  Q_nominal_unit=W
  Thermal Reference : fl_lib/Thermal/Thermal Elements/Thermal Reference
  Battery Conductivity Connection Input : PMIOPort  Side=Left
  Power in : PMIOPort  Port=2  Side=Left
  Water Jacket : PMIOPort  Port=3  Side=Right
  connections:
  Conductive Heat Transfer7/RConn1 -- Conductive Heat Transfer8/LConn1
  Conductive Heat Transfer6/RConn1 -- Conductive Heat Transfer3/LConn1
  Conductive Heat Transfer18/RConn1 -- Conductive Heat Transfer14/RConn1 -- Conductive Heat Transfer10/RConn1 -- Conductive Heat Transfer2/RConn1 -- Conductive Heat Transfer5/RConn1 -- Water Jacket/RConn1
  Conductive Heat Transfer8/RConn1 -- Conductive Heat Transfer10/LConn1 -- Thermal Mass2/LConn1 -- Conductive Heat Transfer9/LConn1 -- Conductive Heat Transfer12/RConn1 -- Thermal Mass3/LConn1 -- Conductive Heat Transfer14/LConn1 -- Conductive Heat Transfer13/LConn1 -- Conductive Heat Transfer18/LConn1 -- Thermal Mass4/LConn1 -- Conductive Heat Transfer16/RConn1 -- Conductive Heat Transfer2/LConn1 -- Thermal Mass/LConn1 -- Conductive Heat Transfer/RConn1 -- Conductive Heat Transfer1/LConn1 -- Conductive Heat Transfer5/LConn1 -- Thermal Mass1/LConn1 -- Conductive Heat Transfer3/RConn1 -- Conductive Heat Transfer4/LConn1 -- Controlled Heat Flow Rate Source/LConn1
  Conductive Heat Transfer15/LConn1 -- Conductive Heat Transfer13/RConn1
  Conductive Heat Transfer11/LConn1 -- Conductive Heat Transfer9/RConn1
  Conductive Heat Transfer7/LConn1 -- Conductive Heat Transfer4/RConn1
  Conductive Heat Transfer11/RConn1 -- Conductive Heat Transfer12/LConn1
  Conductive Heat Transfer6/LConn1 -- Conductive Heat Transfer1/RConn1
  Conductive Heat Transfer15/RConn1 -- Conductive Heat Transfer16/LConn1
  Conductive Heat Transfer/LConn1 -- Battery Conductivity Connection Input/RConn1
  Thermal Reference/LConn1 -- Controlled Heat Flow Rate Source/RConn2
  Dividing Dissipation Bertween Cells/LConn1 -- Power in/RConn1
  Dividing Dissipation Bertween Cells/RConn1 -- Controlled Heat Flow Rate Source/RConn1

== system Model_V5/HVAC/Ext. Forced h/Air Properties ==
  Density Lookup : fl_lib/Physical Signals/Lookup Tables/PS Lookup Table (1D)  x=[-10:1:100] + 273.15 K  f=PropsSI('D','T',([-10:1:100] + 273.15),'P',101325,'AIR') kg/m^3  interp_method=simscape.enum.interpolation.smooth  extrap_method=simscape.enum.extrapolation.linear
  Dynamic Viscosity Lookup : fl_lib/Physical Signals/Lookup Tables/PS Lookup Table (1D)  x=[-10:1:100] + 273.15 K  f=PropsSI('V','T',([-10:1:100] + 273.15),'P',101325,'AIR') Pa*s  interp_method=simscape.enum.interpolation.smooth  extrap_method=simscape.enum.extrapolation.linear
  Prandtl Lookup : fl_lib/Physical Signals/Lookup Tables/PS Lookup Table (1D)  x=[-10:1:100] + 273.15 K  f=PropsSI('PRANDTL','T',([-10:1:100] + 273.15),'P',101325,'AIR')  interp_method=simscape.enum.interpolation.smooth  extrap_method=simscape.enum.extrapolation.linear
  Thermal Conductivity Lookup : fl_lib/Physical Signals/Lookup Tables/PS Lookup Table (1D)  x=[-10:1:100] + 273.15 K  f=PropsSI('L','T',([-10:1:100] + 273.15),'P',101325,'AIR') W/m/K  interp_method=simscape.enum.interpolation.smooth  extrap_method=simscape.enum.extrapolation.linear
  T : PMIOPort  Side=Left
  ρ : PMIOPort  Port=2  Side=Right
  μ : PMIOPort  Port=3  Side=Right
  Pr : PMIOPort  Port=4  Side=Right
  k : PMIOPort  Port=5  Side=Right
  connections:
  Dynamic Viscosity Lookup/RConn1 -- μ/RConn1
  Prandtl Lookup/RConn1 -- Pr/RConn1
  Thermal Conductivity Lookup/RConn1 -- k/RConn1
  Density Lookup/RConn1 -- ρ/RConn1
  Prandtl Lookup/LConn1 -- T/RConn1 -- Thermal Conductivity Lookup/LConn1 -- Dynamic Viscosity Lookup/LConn1 -- Density Lookup/LConn1

== system Model_V5/HVAC/Ext. Forced h/Reynolds Number ==
  "ρv " : fl_lib/Physical Signals/Functions/PS Product
  ρvL : fl_lib/Physical Signals/Functions/PS Gain  gain=10 m
  ρvL/μ : fl_lib/Physical Signals/Functions/PS Divide
  v : PMIOPort  Side=Left
  ρ : PMIOPort  Port=2  Side=Left
  Re : PMIOPort  Port=3  Side=Right
  μ : PMIOPort  Port=4  Side=Left
  connections:
  ρvL/μ/LConn1 -- ρvL/RConn1
  ρvL/μ/RConn1 -- Re/RConn1
  ρvL/LConn1 -- "ρv "/RConn1
  "ρv "/LConn2 -- ρ/RConn1
  "ρv "/LConn1 -- v/RConn1
  ρvL/μ/LConn2 -- μ/RConn1

== system Model_V5/HVAC/Ext. Natural h/Air Properties ==
  Diffusivity Lookup : fl_lib/Physical Signals/Lookup Tables/PS Lookup Table (1D)  x=[-10:1:100] + 273.15 K  f=(PropsSI('L','T',([-10:1:100] + 273.15),'P',101325,'AIR'))./(PropsSI('D','T',([-10:1:100] + 273.15),'P',101325,'AIR'))./(PropsSI('C','T',([-10:1:100] + 273.15),'P',101325,'AIR')) m^2/s  interp_method=simscape.enum.interpolation.smooth  extrap_method=simscape.enum.extrapolation.linear
  Expansion Lookup : fl_lib/Physical Signals/Lookup Tables/PS Lookup Table (1D)  x=[-10:1:100] + 273.15 K  f=PropsSI('ISOBARIC_EXPANSION_COEFFICIENT','T',([-10:1:100] + 273.15),'P',101325,'AIR') 1/K  interp_method=simscape.enum.interpolation.smooth  extrap_method=simscape.enum.extrapolation.linear
  Kinematic Viscosity Lookup : fl_lib/Physical Signals/Lookup Tables/PS Lookup Table (1D)  x=[-10:1:100] + 273.15 K  f=(PropsSI('V','T',([-10:1:100] + 273.15),'P',101325,'AIR'))./(PropsSI('D','T',([-10:1:100] + 273.15),'P',101325,'AIR')) m^2/s  interp_method=simscape.enum.interpolation.smooth  extrap_method=simscape.enum.extrapolation.linear
  Prandtl Lookup : fl_lib/Physical Signals/Lookup Tables/PS Lookup Table (1D)  x=[-10:1:100] + 273.15 K  f=PropsSI('PRANDTL','T',([-10:1:100] + 273.15),'P',101325,'AIR')  interp_method=simscape.enum.interpolation.smooth  extrap_method=simscape.enum.extrapolation.linear
  Thermal Conductivity Lookup : fl_lib/Physical Signals/Lookup Tables/PS Lookup Table (1D)  x=[-10:1:100] + 273.15 K  f=PropsSI('L','T',([-10:1:100] + 273.15),'P',101325,'AIR') W/m/K  interp_method=simscape.enum.interpolation.smooth  extrap_method=simscape.enum.extrapolation.linear
  T : PMIOPort  Side=Left
  β : PMIOPort  Port=2  Side=Right
  α : PMIOPort  Port=3  Side=Right
  ν : PMIOPort  Port=4  Side=Right
  Pr : PMIOPort  Port=5  Side=Right
  k : PMIOPort  Port=6  Side=Right
  connections:
  Thermal Conductivity Lookup/LConn1 -- Prandtl Lookup/LConn1 -- T/RConn1 -- Expansion Lookup/LConn1 -- Kinematic Viscosity Lookup/LConn1 -- Diffusivity Lookup/LConn1
  Thermal Conductivity Lookup/RConn1 -- k/RConn1
  Prandtl Lookup/RConn1 -- Pr/RConn1
  Expansion Lookup/RConn1 -- β/RConn1
  α/RConn1 -- Diffusivity Lookup/RConn1
  ν/RConn1 -- Kinematic Viscosity Lookup/RConn1

== system Model_V5/HVAC/Ext. Natural h/Rayleigh Number ==
  g|∆T| : fl_lib/Physical Signals/Functions/PS Gain  gain=9.8066 m/s^2
  gβ|∆T| : fl_lib/Physical Signals/Functions/PS Product
  gβ|∆T| L³ : fl_lib/Physical Signals/Functions/PS Gain  gain=14^3 ft^3
  gβ|∆T| L³/α : fl_lib/Physical Signals/Functions/PS Divide
  gβ|∆T| L³/α/ν : fl_lib/Physical Signals/Functions/PS Divide
  |∆T| : fl_lib/Physical Signals/Nonlinear Operators/PS Abs
      settings: InternalSimscapePortConfiguration="{\"Bottom\":[],\"Left\":[{\"id\":\"I\",\"label\":\"\",\"type\":\"input\"}],\"Right\":[{\"id\":\"O\",\"label\":\"\",\"type\":\"output\"}],\"Top\":[]}"
  ∆T : fl_lib/Physical Signals/Functions/PS Subtract
  β : PMIOPort  Side=Left
  α : PMIOPort  Port=2  Side=Left
  ν : PMIOPort  Port=3  Side=Left
  Ts : PMIOPort  Port=4  Side=Left
  Tair : PMIOPort  Port=5  Side=Left
  Ra : PMIOPort  Port=6  Side=Right
  connections:
  gβ|∆T| L³/α/LConn1 -- gβ|∆T| L³/RConn1
  gβ|∆T|/LConn1 -- β/RConn1
  gβ|∆T| L³/α/ν/LConn1 -- gβ|∆T| L³/α/RConn1
  g|∆T|/LConn1 -- |∆T|/RConn1
  gβ|∆T|/LConn2 -- g|∆T|/RConn1
  |∆T|/LConn1 -- ∆T/RConn1
  gβ|∆T| L³/LConn1 -- gβ|∆T|/RConn1
  gβ|∆T| L³/α/ν/RConn1 -- Ra/RConn1
  gβ|∆T| L³/α/LConn2 -- α/RConn1
  ∆T/LConn2 -- Tair/RConn1
  ∆T/LConn1 -- Ts/RConn1
  ν/RConn1 -- gβ|∆T| L³/α/ν/LConn2

== system Model_V5/HVAC/HVAC h/Air Properties ==
  Density Lookup : fl_lib/Physical Signals/Lookup Tables/PS Lookup Table (1D)  x=[-10:1:100] + 273.15 K  f=PropsSI('D','T',([-10:1:100] + 273.15),'P',101325,'AIR') kg/m^3  interp_method=simscape.enum.interpolation.smooth  extrap_method=simscape.enum.extrapolation.linear
  Dynamic Viscosity Lookup : fl_lib/Physical Signals/Lookup Tables/PS Lookup Table (1D)  x=[-10:1:100] + 273.15 K  f=PropsSI('V','T',([-10:1:100] + 273.15),'P',101325,'AIR') Pa*s  interp_method=simscape.enum.interpolation.smooth  extrap_method=simscape.enum.extrapolation.linear
  Prandtl Lookup : fl_lib/Physical Signals/Lookup Tables/PS Lookup Table (1D)  x=[-10:1:100] + 273.15 K  f=PropsSI('PRANDTL','T',([-10:1:100] + 273.15),'P',101325,'AIR')  interp_method=simscape.enum.interpolation.smooth  extrap_method=simscape.enum.extrapolation.linear
  Thermal Conductivity Lookup : fl_lib/Physical Signals/Lookup Tables/PS Lookup Table (1D)  x=[-10:1:100] + 273.15 K  f=PropsSI('L','T',([-10:1:100] + 273.15),'P',101325,'AIR') W/m/K  interp_method=simscape.enum.interpolation.smooth  extrap_method=simscape.enum.extrapolation.linear
  T : PMIOPort  Side=Left
  ρ : PMIOPort  Port=2  Side=Right
  μ : PMIOPort  Port=3  Side=Right
  Pr : PMIOPort  Port=4  Side=Right
  k : PMIOPort  Port=5  Side=Right
  connections:
  Dynamic Viscosity Lookup/RConn1 -- μ/RConn1
  Prandtl Lookup/RConn1 -- Pr/RConn1
  Thermal Conductivity Lookup/RConn1 -- k/RConn1
  Density Lookup/RConn1 -- ρ/RConn1
  Prandtl Lookup/LConn1 -- T/RConn1 -- Thermal Conductivity Lookup/LConn1 -- Dynamic Viscosity Lookup/LConn1 -- Density Lookup/LConn1

== system Model_V5/HVAC/HVAC h/Reynolds Number ==
  ρv : fl_lib/Physical Signals/Functions/PS Gain  gain=100 ft/s
  ρvL : fl_lib/Physical Signals/Functions/PS Gain  gain=221*2 in
  ρvL/μ : fl_lib/Physical Signals/Functions/PS Divide
  ρ : PMIOPort  Side=Left
  Re : PMIOPort  Port=2  Side=Right
  μ : PMIOPort  Port=3  Side=Left
  connections:
  ρvL/μ/LConn1 -- ρvL/RConn1
  ρvL/μ/RConn1 -- Re/RConn1
  ρvL/μ/LConn2 -- μ/RConn1
  ρv/RConn1 -- ρvL/LConn1
  ρv/LConn1 -- ρ/RConn1

== system Model_V5/HVAC/Window (Front) h/Air Properties ==
  Diffusivity Lookup : fl_lib/Physical Signals/Lookup Tables/PS Lookup Table (1D)  x=[-10:1:100] + 273.15 K  f=(PropsSI('L','T',([-10:1:100] + 273.15),'P',101325,'AIR'))./(PropsSI('D','T',([-10:1:100] + 273.15),'P',101325,'AIR'))./(PropsSI('C','T',([-10:1:100] + 273.15),'P',101325,'AIR')) m^2/s  interp_method=simscape.enum.interpolation.smooth  extrap_method=simscape.enum.extrapolation.linear
  Expansion Lookup : fl_lib/Physical Signals/Lookup Tables/PS Lookup Table (1D)  x=[-10:1:100] + 273.15 K  f=PropsSI('ISOBARIC_EXPANSION_COEFFICIENT','T',([-10:1:100] + 273.15),'P',101325,'AIR') 1/K  interp_method=simscape.enum.interpolation.smooth  extrap_method=simscape.enum.extrapolation.linear
  Kinematic Viscosity Lookup : fl_lib/Physical Signals/Lookup Tables/PS Lookup Table (1D)  x=[-10:1:100] + 273.15 K  f=(PropsSI('V','T',([-10:1:100] + 273.15),'P',101325,'AIR'))./(PropsSI('D','T',([-10:1:100] + 273.15),'P',101325,'AIR')) m^2/s  interp_method=simscape.enum.interpolation.smooth  extrap_method=simscape.enum.extrapolation.linear
  Prandtl Lookup : fl_lib/Physical Signals/Lookup Tables/PS Lookup Table (1D)  x=[-10:1:100] + 273.15 K  f=PropsSI('PRANDTL','T',([-10:1:100] + 273.15),'P',101325,'AIR')  interp_method=simscape.enum.interpolation.smooth  extrap_method=simscape.enum.extrapolation.linear
  Thermal Conductivity Lookup : fl_lib/Physical Signals/Lookup Tables/PS Lookup Table (1D)  x=[-10:1:100] + 273.15 K  f=PropsSI('L','T',([-10:1:100] + 273.15),'P',101325,'AIR') W/m/K  interp_method=simscape.enum.interpolation.smooth  extrap_method=simscape.enum.extrapolation.linear
  T : PMIOPort  Side=Left
  β : PMIOPort  Port=2  Side=Right
  α : PMIOPort  Port=3  Side=Right
  ν : PMIOPort  Port=4  Side=Right
  Pr : PMIOPort  Port=5  Side=Right
  k : PMIOPort  Port=6  Side=Right
  connections:
  Thermal Conductivity Lookup/LConn1 -- Prandtl Lookup/LConn1 -- T/RConn1 -- Expansion Lookup/LConn1 -- Kinematic Viscosity Lookup/LConn1 -- Diffusivity Lookup/LConn1
  Thermal Conductivity Lookup/RConn1 -- k/RConn1
  Prandtl Lookup/RConn1 -- Pr/RConn1
  Expansion Lookup/RConn1 -- β/RConn1
  α/RConn1 -- Diffusivity Lookup/RConn1
  ν/RConn1 -- Kinematic Viscosity Lookup/RConn1

== system Model_V5/HVAC/Window (Front) h/Rayleigh Number ==
  note: For inclined plate, g = g*cos θ
  g|∆T| : fl_lib/Physical Signals/Functions/PS Gain  gain=9.8066*0.5 m/s^2
  gβ|∆T| : fl_lib/Physical Signals/Functions/PS Product
  gβ|∆T| L³ : fl_lib/Physical Signals/Functions/PS Gain  gain=14^3 ft^3
  gβ|∆T| L³/α : fl_lib/Physical Signals/Functions/PS Divide
  gβ|∆T| L³/α/ν : fl_lib/Physical Signals/Functions/PS Divide
  |∆T| : fl_lib/Physical Signals/Nonlinear Operators/PS Abs
      settings: InternalSimscapePortConfiguration="{\"Bottom\":[],\"Left\":[{\"id\":\"I\",\"label\":\"\",\"type\":\"input\"}],\"Right\":[{\"id\":\"O\",\"label\":\"\",\"type\":\"output\"}],\"Top\":[]}"
  ∆T : fl_lib/Physical Signals/Functions/PS Subtract
  β : PMIOPort  Side=Left
  α : PMIOPort  Port=2  Side=Left
  ν : PMIOPort  Port=3  Side=Left
  Ts : PMIOPort  Port=4  Side=Left
  Tair : PMIOPort  Port=5  Side=Left
  Ra : PMIOPort  Port=6  Side=Right
  connections:
  gβ|∆T| L³/α/LConn1 -- gβ|∆T| L³/RConn1
  gβ|∆T|/LConn1 -- β/RConn1
  gβ|∆T| L³/α/ν/LConn1 -- gβ|∆T| L³/α/RConn1
  g|∆T|/LConn1 -- |∆T|/RConn1
  gβ|∆T|/LConn2 -- g|∆T|/RConn1
  |∆T|/LConn1 -- ∆T/RConn1
  gβ|∆T| L³/LConn1 -- gβ|∆T|/RConn1
  gβ|∆T| L³/α/ν/RConn1 -- Ra/RConn1
  gβ|∆T| L³/α/LConn2 -- α/RConn1
  ∆T/LConn2 -- Tair/RConn1
  ∆T/LConn1 -- Ts/RConn1
  ν/RConn1 -- gβ|∆T| L³/α/ν/LConn2

== system Model_V5/HVAC/Window (Side) h/Air Properties ==
  Diffusivity Lookup : fl_lib/Physical Signals/Lookup Tables/PS Lookup Table (1D)  x=[-10:1:100] + 273.15 K  f=(PropsSI('L','T',([-10:1:100] + 273.15),'P',101325,'AIR'))./(PropsSI('D','T',([-10:1:100] + 273.15),'P',101325,'AIR'))./(PropsSI('C','T',([-10:1:100] + 273.15),'P',101325,'AIR')) m^2/s  interp_method=simscape.enum.interpolation.smooth  extrap_method=simscape.enum.extrapolation.linear
  Expansion Lookup : fl_lib/Physical Signals/Lookup Tables/PS Lookup Table (1D)  x=[-10:1:100] + 273.15 K  f=PropsSI('ISOBARIC_EXPANSION_COEFFICIENT','T',([-10:1:100] + 273.15),'P',101325,'AIR') 1/K  interp_method=simscape.enum.interpolation.smooth  extrap_method=simscape.enum.extrapolation.linear
  Kinematic Viscosity Lookup : fl_lib/Physical Signals/Lookup Tables/PS Lookup Table (1D)  x=[-10:1:100] + 273.15 K  f=(PropsSI('V','T',([-10:1:100] + 273.15),'P',101325,'AIR'))./(PropsSI('D','T',([-10:1:100] + 273.15),'P',101325,'AIR')) m^2/s  interp_method=simscape.enum.interpolation.smooth  extrap_method=simscape.enum.extrapolation.linear
  Prandtl Lookup : fl_lib/Physical Signals/Lookup Tables/PS Lookup Table (1D)  x=[-10:1:100] + 273.15 K  f=PropsSI('PRANDTL','T',([-10:1:100] + 273.15),'P',101325,'AIR')  interp_method=simscape.enum.interpolation.smooth  extrap_method=simscape.enum.extrapolation.linear
  Thermal Conductivity Lookup : fl_lib/Physical Signals/Lookup Tables/PS Lookup Table (1D)  x=[-10:1:100] + 273.15 K  f=PropsSI('L','T',([-10:1:100] + 273.15),'P',101325,'AIR') W/m/K  interp_method=simscape.enum.interpolation.smooth  extrap_method=simscape.enum.extrapolation.linear
  T : PMIOPort  Side=Left
  β : PMIOPort  Port=2  Side=Right
  α : PMIOPort  Port=3  Side=Right
  ν : PMIOPort  Port=4  Side=Right
  Pr : PMIOPort  Port=5  Side=Right
  k : PMIOPort  Port=6  Side=Right
  connections:
  T/RConn1 -- Thermal Conductivity Lookup/LConn1 -- Prandtl Lookup/LConn1 -- Expansion Lookup/LConn1 -- Kinematic Viscosity Lookup/LConn1 -- Diffusivity Lookup/LConn1
  Thermal Conductivity Lookup/RConn1 -- k/RConn1
  Prandtl Lookup/RConn1 -- Pr/RConn1
  Expansion Lookup/RConn1 -- β/RConn1
  α/RConn1 -- Diffusivity Lookup/RConn1
  ν/RConn1 -- Kinematic Viscosity Lookup/RConn1
